simulink model "naolinear"  (R2015a)
settings: Solver=ode45  StartTime=0.0  StopTime=200  RelTol=1e-3
values from neighbouring files (symbols this model uses):
  B = 0.1    [AT1.m]
  J = 1    [AT1.m]
  Kw = 1/3    (= 0.333333333333)    [AT1.m]
  L = 0.5    [AT1.m]
  R = 10    [AT1.m]
settings Model: Creator=guilh  LastModifiedBy=guilh

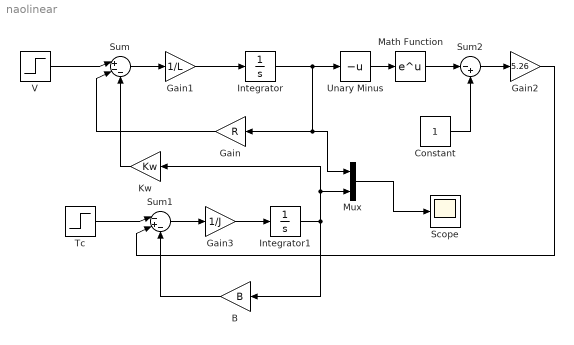
== system naolinear ==
  B : Gain  Gain=B
  Constant : Constant
  Gain : Gain  Gain=R
  Gain1 : Gain  Gain=1/L
  Gain2 : Gain  Gain=5.26
  Gain3 : Gain  Gain=1/J
  Integrator : Integrator
  Integrator1 : Integrator
  Kw : Gain  Gain=Kw
  Math Function : Math  SaturateOnIntegerOverflow=on
  Mux : Mux  Inputs=2
  Scope : Scope
  Sum : Sum  Inputs=|+--
  Sum1 : Sum  Inputs=|-+-
  Sum2 : Sum  Inputs=|-+
  Tc : Step  Time=100  SampleTime=0
  Unary Minus : UnaryMinus
  V : Step  Time=0  After=30  SampleTime=0
  wires:
  V/1 -> Sum/1
  Gain/1 -> Sum/2
  Integrator/1 -> Unary Minus/1, Mux/1, Gain/1
  Sum/1 -> Gain1/1
  Gain1/1 -> Integrator/1
  Kw/1 -> Sum/3
  Tc/1 -> Sum1/1
  Gain3/1 -> Integrator1/1
  Sum1/1 -> Gain3/1
  Integrator1/1 -> Mux/2, Kw/1, B/1
  B/1 -> Sum1/3
  Unary Minus/1 -> Math Function/1
  Math Function/1 -> Sum2/1
  Constant/1 -> Sum2/2
  Sum2/1 -> Gain2/1
  Gain2/1 -> Sum1/2
  Mux/1 -> Scope/1
